simulink model "twoLFCmodlenew_25"  (R2021a)
settings: Solver=ode45  StartTime=0.0  StopTime=5  FixedStep=1e-2  RelTol=1e-3  EnableMultiTasking=on
values from neighbouring files (symbols this model uses):
  Kd1 = 15.9765642389    [GBOFOPID.mat]    (also in GBOPID.mat = 25.4175594756)
  Kd2 = 16.1555667572    [GBOFOPID.mat]    (also in GBOPID.mat = 16.5820539589)
  Ki1 = 519.767648526    [GBOFOPID.mat]    (also in GBOPID.mat = 385.334235788)
  Ki2 = 683.657    [GBOFOPID.mat]    (also in GBOPID.mat = 430.561364416)
  Kp1 = 385.424894233    [GBOFOPID.mat]    (also in GBOPID.mat = 68.2193459651)
  Kp2 = 695.178644613    [GBOFOPID.mat]    (also in GBOPID.mat = 61.772896549)
libraries: fod x2
settings Model: Creator=kiran.kulkarni  LastModifiedBy=wp
settings SolverCC: ZeroCrossAlgorithm=Adaptive  AlgebraicLoopSolver=TrustRegion
settings DataIOCC: SaveFormat=Array  SignalLoggingSaveFormat=ModelDataLogs  ReturnWorkspaceOutputs=off
settings OptimizationCC: ExpressionDepthLimit=2147483647  InitFltsAndDblsToZero=on  LifeSpan=inf
settings DebuggingCC: SaveWithParameterizedLinksMsg=none  UnderspecifiedInitializationDetection=Classic  MergeDetectMultiDrivingBlocksExec=none  SignalResolutionControl=TryResolveAllWithWarning  MaskedZcDiagnostic=none  IgnoredZcDiagnostic=none  MultiTaskDSMMsg=warning  MultiTaskCondExecSysMsg=none  FcnCallInpInsideContextMsg=warning  StateNameClashWarn=warning  SFUnexpectedBacktrackingDiag=warning  SFNoUnconditionalDefaultTransitionDiag=warning  SFExecutionAtInitializationDiag=none  SFMachineParentedDataDiag=warning  ArithmeticOperatorsInVariantConditions=warning
settings HardwareCC: ProdBitPerPointer=32  ProdBitPerSizeT=32  ProdBitPerPtrDiffT=32  ProdLargestAtomicFloat=None  ProdIntDivRoundTo=Undefined  ProdEndianess=Unspecified  ProdWordSize=32  ProdHWDeviceType=32-bit Generic
settings ModelReferenceCC: PropagateSignalLabelsOutOfModel=off
settings SFSimCC: SimUseLocalCustomCode=off  CustomCodeUndefinedFunction=UseInterfaceOnly
settings RTWCC: RTWUseLocalCustomCode=off
settings CodeAppCC: StateflowObjectComments=on
settings GRTTargetCC: TargetFcnLib=ansi_tfl_tmw.mat  TargetLangStandard=C89/C90 (ANSI)  CombineOutputUpdateFcns=off  GRTInterface=on
settings ConfigComp: CovMetricSettings=dw  CovSaveCumulativeToWorkspaceVar=on  CovSaveSingleToWorkspaceVar=on  CovExternalEMLEnable=off

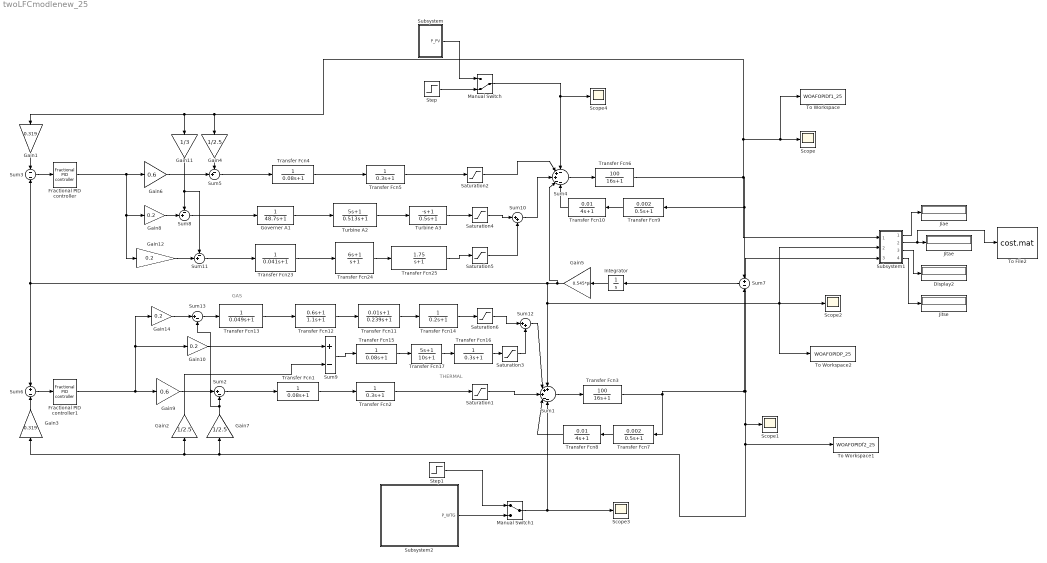
== system twoLFCmodlenew_25 ==
  note: GAS
  note: THERMAL
  Display2 : Display
  Fractional PID controller : fod/Fractional PID controller  Kp=Kp1  Ki=Ki1  lambda=lam1  Kd=Kd1  mic=mu1  freqRange=[0.001, 1000]  N=5
      link override Fractional derivative1: nFod=on
      link override Fractional integrator1: nFod=on
      settings: SourceProductName=FOMCON Toolbox
  Fractional PID controller1 : fod/Fractional PID controller  Kp=Kp2  Ki=Ki2  lambda=lam2  Kd=Kd2  mic=mu2  freqRange=[0.001, 1000]  N=5
      link override Fractional derivative1: nFod=on
      link override Fractional integrator1: nFod=on
      settings: SourceProductName=FOMCON Toolbox
  Gain1 : Gain  Gain=0.319
  Gain{8,10,12,14} (4 alike) : Gain  Gain=0.2
  Gain11 : Gain  Gain=1/3
  Gain2 : Gain  Gain=1/2.5
  Gain3 : Gain  Gain=0.319
  Gain4 : Gain  Gain=1/2.5
  Gain5 : Gain  Gain=0.545*pi
  Gain6 : Gain  Gain=0.6
  Gain7 : Gain  Gain=1/2.5
  Gain9 : Gain  Gain=0.6
  Governer A1 : TransferFcn  Denominator=[48.7 1]
  Integrator : Integrator
  Jiae : Display
  Jitae : Display
  Jitse : Display
  Manual Switch : ManualSwitch  CurrentSetting=0
  Manual Switch1 : ManualSwitch
  Saturation{1..6} (6 alike) : Saturate  UpperLimit=0.1  LowerLimit=-0.1
  Scope{,1..4} (5 alike) : Scope
  Step : Step  Time=0  After=0.01  SampleTime=0
  Step1 : Step  Time=0  After=0.01  SampleTime=0
  Subsystem : Subsystem
  Subsystem1 : Subsystem
  Subsystem2 : Subsystem
  Sum1 : Sum  Inputs=+++--
  Sum10 : Sum  Inputs=|++
  Sum11 : Sum  Inputs=-+|
  Sum12 : Sum  Inputs=|++
  Sum13 : Sum  Inputs=|+-
  Sum2 : Sum  Inputs=|+-
  Sum3 : Sum  Inputs=--
  Sum4 : Sum  Inputs=-++--
  Sum5 : Sum  Inputs=-+|
  Sum6 : Sum  Inputs=+-
  Sum7 : Sum  Inputs=+-
  Sum8 : Sum  Inputs=-+|
  Sum9 : Sum  Inputs=+-
  To File2 : ToFile  Filename=cost.mat  MatrixName=cost
  To Workspace : ToWorkspace  VariableName=WOAFOPIDf1_25  SaveFormat=Timeseries  SampleTime=-1
  To Workspace1 : ToWorkspace  VariableName=WOAFOPIDf2_25  SaveFormat=Timeseries  SampleTime=-1
  To Workspace2 : ToWorkspace  VariableName=WOAFOPIDP_25  SaveFormat=Timeseries  SampleTime=-1
  Transfer Fcn1 : TransferFcn  Denominator=[0.08 1]
  Transfer Fcn10 : TransferFcn  Numerator=[0.01]  Denominator=[4 1]
  Transfer Fcn11 : TransferFcn  Numerator=[0.01 1]  Denominator=[0.239 1]
  Transfer Fcn12 : TransferFcn  Numerator=[0.6 1]  Denominator=[1.1 1]
  Transfer Fcn13 : TransferFcn  Denominator=[0.049 1]
  Transfer Fcn14 : TransferFcn  Numerator=[ 1]  Denominator=[0.2 1]
  Transfer Fcn15 : TransferFcn  Denominator=[0.08 1]
  Transfer Fcn16 : TransferFcn  Denominator=[0.3 1]
  Transfer Fcn17 : TransferFcn  Numerator=[5 1]  Denominator=[10 1]
  Transfer Fcn2 : TransferFcn  Denominator=[0.3 1]
  Transfer Fcn23 : TransferFcn  Denominator=[0.041 1]
  Transfer Fcn24 : TransferFcn  Numerator=[6 1]  Denominator=[1 1]
  Transfer Fcn25 : TransferFcn  Numerator=[0 1.75]  Denominator=[1 1]
  Transfer Fcn3 : TransferFcn  Numerator=[100]  Denominator=[16 1]
  Transfer Fcn4 : TransferFcn  Denominator=[0.08 1]
  Transfer Fcn5 : TransferFcn  Denominator=[0.3 1]
  Transfer Fcn6 : TransferFcn  Numerator=[100]  Denominator=[16 1]
  Transfer Fcn7 : TransferFcn  Numerator=[0.002]  Denominator=[0.5 1]
  Transfer Fcn8 : TransferFcn  Numerator=[0.01]  Denominator=[4 1]
  Transfer Fcn9 : TransferFcn  Numerator=[0.002]  Denominator=[0.5 1]
  Turbine A2 : TransferFcn  Numerator=[5 1]  Denominator=[0.513 1]
  Turbine A3 : TransferFcn  Numerator=[-1 1]  Denominator=[0.5 1]
  wires:
  Sum4/1 -> Transfer Fcn6/1
  Transfer Fcn1/1 -> Transfer Fcn2/1
  Sum1/1 -> Transfer Fcn3/1
  Gain1/1 -> Sum3/1
  Gain2/1 -> Sum9/2
  Sum6/1 -> Fractional PID controller1/1
  Gain3/1 -> Sum6/2
  Sum7/1 -> Integrator/1
  Integrator/1 -> Gain5/1
  Subsystem1/1(Jiae) -> Jiae/1
  Subsystem1/2(Jitae) -> To File2/1, Jitae/1
  Subsystem1/4(Jitse) -> Jitse/1
  Transfer Fcn6/1 -> Sum7/1, Transfer Fcn9/1, To Workspace/1, Scope/1, Gain1/1, Gain11/1, Gain4/1, Subsystem1/1(Input)
  Subsystem1/3(Jise) -> Display2/1
  Gain4/1 -> Sum5/1
  Gain7/1 -> Sum13/2, Sum2/2
  Sum9/1 -> Transfer Fcn15/1
  Saturation3/1 -> Sum12/2
  Transfer Fcn16/1 -> Saturation3/1
  Transfer Fcn7/1 -> Transfer Fcn8/1
  Transfer Fcn9/1 -> Transfer Fcn10/1
  Transfer Fcn3/1 -> Subsystem1/3(Input2), To Workspace1/1, Gain7/1, Gain3/1, Gain2/1, Scope1/1, Sum7/2, Transfer Fcn7/1
  Fractional PID controller1/1 -> Gain9/1, Gain14/1, Gain10/1
  Turbine A3/1 -> Saturation4/1
  Saturation4/1 -> Sum10/1
  Gain6/1 -> Sum5/2
  Gain8/1 -> Sum8/2
  Gain9/1 -> Sum2/1
  Gain10/1 -> Sum9/1
  Gain11/1 -> Sum11/1, Sum8/1
  Sum8/1 -> Governer A1/1
  Governer A1/1 -> Turbine A2/1
  Turbine A2/1 -> Turbine A3/1
  Gain5/1 -> Sum4/4, Sum6/1, Sum3/2, To Workspace2/1, Subsystem1/2(Input1), Scope2/1, Sum1/1
  Step/1 -> Manual Switch/2
  Subsystem/1(P_PV) -> Manual Switch/1
  Manual Switch/1 -> Scope4/1, Sum4/1
  Step1/1 -> Manual Switch1/1
  Subsystem2/1(P_WTG) -> Manual Switch1/2
  Manual Switch1/1 -> Scope3/1, Sum1/5
  Transfer Fcn8/1 -> Sum1/4
  Transfer Fcn10/1 -> Sum4/5
  Sum3/1 -> Fractional PID controller/1
  Transfer Fcn25/1 -> Saturation5/1
  Transfer Fcn23/1 -> Transfer Fcn24/1
  Transfer Fcn24/1 -> Transfer Fcn25/1
  Fractional PID controller/1 -> Gain12/1, Gain8/1, Gain6/1
  Gain12/1 -> Sum11/2
  Saturation5/1 -> Sum10/2
  Sum10/1 -> Sum4/3
  Transfer Fcn14/1 -> Saturation6/1
  Transfer Fcn11/1 -> Transfer Fcn14/1
  Gain14/1 -> Sum13/1
  Transfer Fcn12/1 -> Transfer Fcn11/1
  Transfer Fcn13/1 -> Transfer Fcn12/1
  Sum11/1 -> Transfer Fcn23/1
  Saturation6/1 -> Sum12/1
  Sum12/1 -> Sum1/2
  Transfer Fcn17/1 -> Transfer Fcn16/1
  Transfer Fcn15/1 -> Transfer Fcn17/1
  Sum2/1 -> Transfer Fcn1/1
  Transfer Fcn2/1 -> Saturation1/1
  Saturation1/1 -> Sum1/3
  Transfer Fcn4/1 -> Transfer Fcn5/1
  Sum5/1 -> Transfer Fcn4/1
  Transfer Fcn5/1 -> Saturation2/1
  Saturation2/1 -> Sum4/2
  Sum13/1 -> Transfer Fcn13/1

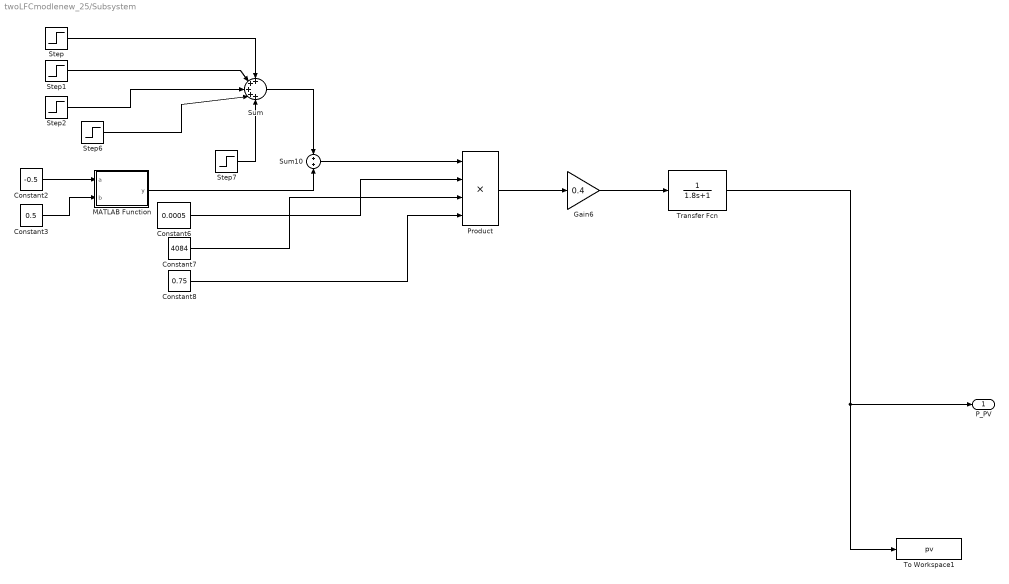
== system twoLFCmodlenew_25/Subsystem ==
  Constant2 : Constant  Value=-0.5
  Constant3 : Constant  Value=0.5
  Constant6 : Constant  Value=0.0005
  Constant7 : Constant  Value=4084
  Constant8 : Constant  Value=0.75
  Gain6 : Gain  Gain=0.4
  MATLAB Function : MATLAB Function  TreatAsAtomicUnit=on
  Product : Product  Inputs=4
  Step : Step  Time=0  After=0.054  SampleTime=0
  Step1 : Step  Time=18  After=0.052  SampleTime=0
  Step2 : Step  Time=37  After=0.028  SampleTime=0
  Step6 : Step  Time=58  After=-0.047  SampleTime=0
  Step7 : Step  Time=74  After=-0.042  SampleTime=0
  Sum : Sum  Inputs=+++++
  Sum10 : Sum
  To Workspace1 : ToWorkspace  VariableName=pv  SaveFormat=Timeseries  SampleTime=-1
  Transfer Fcn : TransferFcn  Denominator=[1.8 1]
  P_PV : Outport
  wires:
  Constant7/1 -> Product/3
  Constant3/1 -> MATLAB Function/2(b)
  Sum/1 -> Sum10/1
  Step7/1 -> Sum/5
  Sum10/1 -> Product/1
  Step2/1 -> Sum/3
  Product/1 -> Gain6/1
  MATLAB Function/1(y) -> Sum10/2
  Constant6/1 -> Product/2
  Step6/1 -> Sum/4
  Step/1 -> Sum/1
  Constant8/1 -> Product/4
  Step1/1 -> Sum/2
  Constant2/1 -> MATLAB Function/1(a)
  Transfer Fcn/1 -> To Workspace1/1, P_PV/1
  Gain6/1 -> Transfer Fcn/1

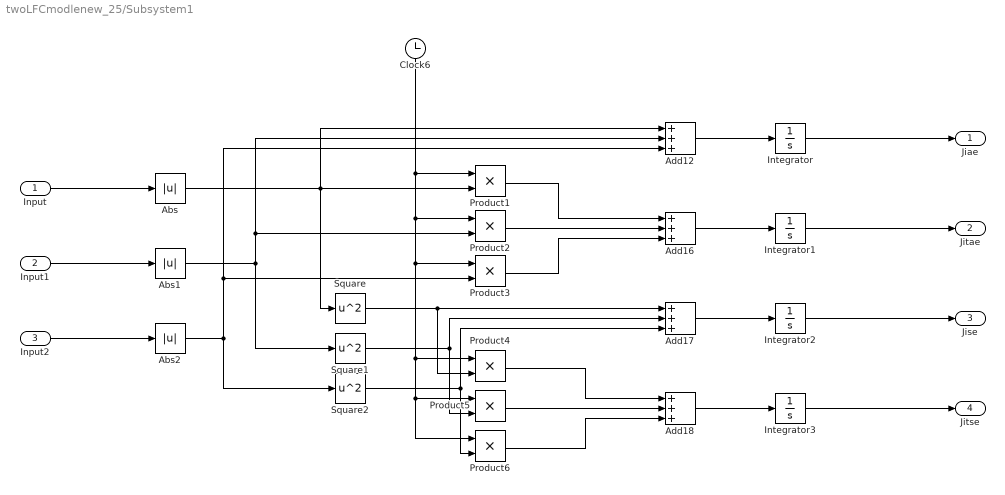
== system twoLFCmodlenew_25/Subsystem1 ==
  Input : Inport
  Input1 : Inport  Port=2
  Input2 : Inport  Port=3
  Abs : Abs
  Abs1 : Abs
  Abs2 : Abs
  Add{12,16..18} (4 alike) : Sum  Inputs=+++
  Clock6 : Clock
  Integrator{,1..3} (4 alike) : Integrator
  Product{1..6} (6 alike) : Product
  Square : Math  Operator=square  SignedPower=on  SaturateOnIntegerOverflow=on
  Square1 : Math  Operator=square  SignedPower=on  SaturateOnIntegerOverflow=on
  Square2 : Math  Operator=square  SignedPower=on  SaturateOnIntegerOverflow=on
  Jiae : Outport  VectorParamsAs1DForOutWhenUnconnected=off
  Jitae : Outport  Port=2  VectorParamsAs1DForOutWhenUnconnected=off
  Jise : Outport  Port=3  VectorParamsAs1DForOutWhenUnconnected=off
  Jitse : Outport  Port=4  VectorParamsAs1DForOutWhenUnconnected=off
  wires:
  Input/1 -> Abs/1
  Product2/1 -> Add16/2
  Integrator1/1 -> Jitae/1
  Clock6/1 -> Product1/1, Product2/1, Product3/1, Product6/1, Product5/1, Product4/1
  Add16/1 -> Integrator1/1
  Integrator/1 -> Jiae/1
  Integrator2/1 -> Jise/1
  Integrator3/1 -> Jitse/1
  Product5/1 -> Add18/2
  Add18/1 -> Integrator3/1
  Add12/1 -> Integrator/1
  Input2/1 -> Abs2/1
  Square/1 -> Add17/1, Product4/2
  Product3/1 -> Add16/3
  Product6/1 -> Add18/3
  Input1/1 -> Abs1/1
  Square2/1 -> Add17/3, Product6/2
  Square1/1 -> Add17/2, Product5/2
  Product1/1 -> Add16/1
  Add17/1 -> Integrator2/1
  Product4/1 -> Add18/1
  Abs/1 -> Square/1, Add12/1, Product1/2
  Abs1/1 -> Add12/2, Product2/2, Square1/1
  Abs2/1 -> Square2/1, Add12/3, Product3/2

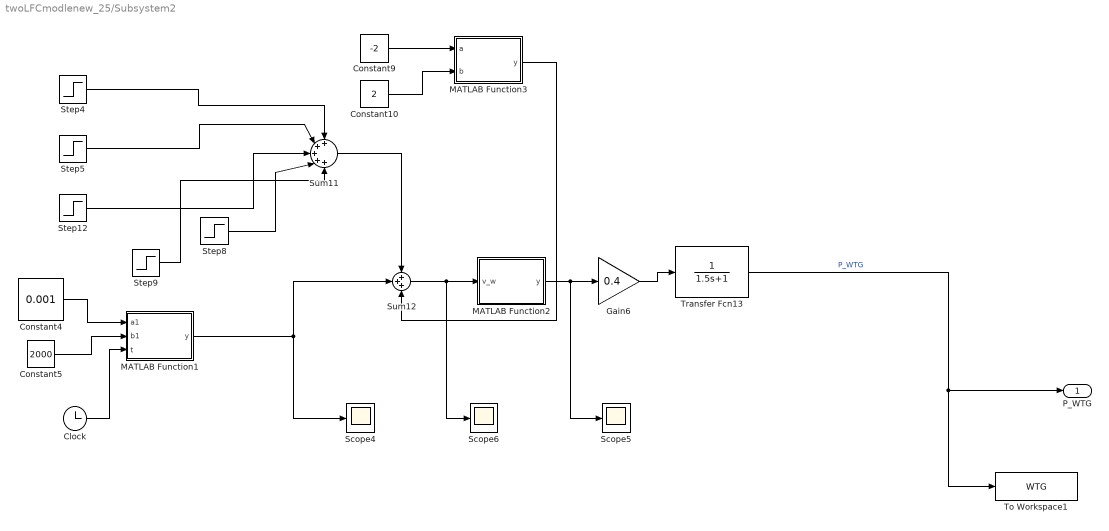
== system twoLFCmodlenew_25/Subsystem2 ==
  Clock : Clock
  Constant10 : Constant  Value=2
  Constant4 : Constant  Value=0.001
  Constant5 : Constant  Value=2000
  Constant9 : Constant  Value=-2
  Gain6 : Gain  Gain=0.4
  MATLAB Function1 : MATLAB Function  TreatAsAtomicUnit=on
  MATLAB Function2 : MATLAB Function  TreatAsAtomicUnit=on
  MATLAB Function3 : MATLAB Function  TreatAsAtomicUnit=on
  Scope4 : Scope
  Scope5 : Scope
  Scope6 : Scope
  Step12 : Step  Time=33  After=-1.1  SampleTime=0
  Step4 : Step  Time=0  After=7.2  SampleTime=0
  Step5 : Step  Time=15  After=-1.4  SampleTime=0
  Step8 : Step  Time=57  After=1.6  SampleTime=0
  Step9 : Step  Time=76  After=1.4  SampleTime=0
  Sum11 : Sum  Inputs=+++++
  Sum12 : Sum  Inputs=+++
  To Workspace1 : ToWorkspace  VariableName=WTG  SaveFormat=Timeseries  SampleTime=-1
  Transfer Fcn13 : TransferFcn  Denominator=[1.5 1]
  P_WTG : Outport
  wires:
  MATLAB Function2/1(y) -> Scope5/1, Gain6/1
  Constant10/1 -> MATLAB Function3/2(b)
  Step12/1 -> Sum11/3
  MATLAB Function1/1(y) -> Scope4/1, Sum12/2
  Step8/1 -> Sum11/4
  Constant9/1 -> MATLAB Function3/1(a)
  Sum11/1 -> Sum12/1
  Step9/1 -> Sum11/5
  Sum12/1 -> Scope6/1, MATLAB Function2/1(v_w)
  Constant5/1 -> MATLAB Function1/2(b1)
  Clock/1 -> MATLAB Function1/3(t)
  Constant4/1 -> MATLAB Function1/1(a1)
  Step5/1 -> Sum11/2
  Step4/1 -> Sum11/1
  MATLAB Function3/1(y) -> Sum12/3
  Transfer Fcn13/1 -> To Workspace1/1, P_WTG/1  "P_WTG"
  Gain6/1 -> Transfer Fcn13/1

== matlab function twoLFCmodlenew_25/Subsystem2/MATLAB Function3 ==
  data: a input; y output; b input
function y = fcn(a,b)

   u1 = a + (b-a) * rand(1,1); 

y = u1;

== matlab function twoLFCmodlenew_25/Subsystem/MATLAB Function ==
  data: a input; y output; b input
function y = fcn(a,b)

   u1 = a + (b-a) * rand(1,1); 

y = u1;

== matlab function twoLFCmodlenew_25/Subsystem2/MATLAB Function1 ==
  settings: updateMethod=DISCRETE
  data: a1 input; y output; b1 input; t input
function y = fcn(a1,b1,t)
   for  i = 1:50
     f_i = 0 + (2*pi-0)*rand;
     w_i = (i-5)*0.5;
     s_v = (2*a1*b1^2*w_i)/(pi^2*(1+((b1*w_i)/(7.5*pi))^2)^(4/3));  
   end
    v_w = 2*4*sum((s_v*0.5)^0.5*cos(w_i*10*t+f_i));
y = v_w;

== matlab function twoLFCmodlenew_25/Subsystem2/MATLAB Function2 ==
  data: v_w input; y output
function y = fcn(v_w)
   lam = 23.5*3.14/v_w; 
   c_p = (0.44-0.0167*0.1745)*sin((pi*(lam-3))/(15-0.3*0.1745))-0.0184*0.1745*(lam-3);
   p_w = 0.0000005*1.25*1735*c_p*v_w^3;
y = p_w;
